simulink model "initial_setup"  (R2012b)
settings: Solver=FixedStepDiscrete  StartTime=0.0  StopTime=inf  FixedStep=sample_time  RelTol=1e-3
InitFcn:
  | init_initial_setup;
values from neighbouring files (symbols this model uses):
  fcut_unwrap = 50    [init_initial_setup.m]
  fcut_velocity = 100    [init_initial_setup.m]
  sample_time = 1/update_freq    (= 0.001)    [init_initial_setup.m]
undefined symbols (not defined in the file or in its folder): A_angle_h, A_angle_k, A_angle_lat, angle_midpoint_h, angle_midpoint_k, angle_midpoint_lat, BOOM_MAX_ENCODER_TICKS, BOOM_PITCH_CAL_VALUE_RAD, BOOM_PITCH_CAL_VALUE_TICKS, BOOM_PITCH_ENCODER_RAD_PER_TICK, BOOM_ROLL_CAL_VALUE_RAD, BOOM_ROLL_CAL_VALUE_TICKS, BOOM_ROLL_ENCODER_RAD_PER_TICK, BOOM_YAW_ENCODER_RAD_PER_TICK, control_start_time, HIP_ABS_ENCODER_RAD_PER_TICK, HIP_INC_ENCODER_RAD_PER_TICK, HIP_INC_MAX_ENCODER_TICKS, k_leg_spring, kd_h_sine_walk, kd_k_sine_walk, kd_lat, kd_sea_position, kd_sea_torque, kd_velocity, kp_h_sine_walk, kp_k_sine_walk, kp_lat, kp_sea_position, kp_sea_torque, kp_velocity, LEFT_HIP_CALIB_POS, LEFT_HIP_CALIB_VAL, LEFT_MOTOR_HIP_DIRECTION, LEG1_LEG_A_CALIB_VAL, LEG1_LEG_A_RAD_PER_CNT, LEG1_LEG_B_CALIB_VAL, LEG1_LEG_B_RAD_PER_CNT, LEG1_MOTOR_A_DIRECTION, LEG1_MOTOR_B_DIRECTION, LEG1_TRAN_A_CALIB_VAL, LEG1_TRAN_A_RAD_PER_CNT, LEG1_TRAN_B_CALIB_VAL, LEG1_TRAN_B_RAD_PER_CNT, LEG2_LEG_A_CALIB_VAL, LEG2_LEG_A_RAD_PER_CNT, LEG2_LEG_B_CALIB_VAL, LEG2_LEG_B_RAD_PER_CNT, LEG2_MOTOR_A_DIRECTION, LEG2_MOTOR_B_DIRECTION, LEG2_TRAN_A_CALIB_VAL, LEG2_TRAN_A_RAD_PER_CNT, LEG2_TRAN_B_CALIB_VAL, LEG2_TRAN_B_RAD_PER_CNT, LEG_A_CALIB_LOC, LEG_B_CALIB_LOC, LEG_MTR_GEAR_RATIO, LEG_MTR_MAX_TORQUE, LEG_MTR_MAX_VELOCITY, MTR_HIP_MAX_CURRENT ... (+10)
libraries: xpcethercatlib x160, simulink x34, dspswit3 x1
(part 4 of 4)

== system initial_setup/Simple Sinusoidal Motion/SEA Controllers (Left Leg)/SEA Controller (Velocity) front/PID/filtered_derivative ==
  x : Inport
  Gain1 : Gain  Gain=1/sample_time
  difference : simulink/Discrete/Difference  ICPrevInput=0.0  InputProcessing=Inherited  OutMin=[]  OutMax=[]  OutDataType=fixdt(1, 16)  OutScaling=2^-10  DoSatur=off
  single_pole_filter : DiscreteTransferFcn  Numerator=[(1-exp(-2*pi*fcut_velocity*sample_time)) 0]  Denominator=[1 -exp(-2*pi*fcut_velocity*sample_time)]  SampleTime=sample_time
  dx/dt : Outport
  wires:
  Gain1/1 -> single_pole_filter/1
  difference/1 -> Gain1/1
  single_pole_filter/1 -> dx/dt/1
  x/1 -> difference/1

== system initial_setup/Simple Sinusoidal Motion/SEA Controllers (Right Leg)/SEA Controller (Position) back/Position PD/filtered_derivative ==
  x : Inport
  Gain1 : Gain  Gain=1/sample_time
  difference : simulink/Discrete/Difference  ICPrevInput=0.0  InputProcessing=Inherited  OutMin=[]  OutMax=[]  OutDataType=fixdt(1, 16)  OutScaling=2^-10  DoSatur=off
  single_pole_filter : DiscreteTransferFcn  Numerator=[(1-exp(-2*pi*fcut_velocity*sample_time)) 0]  Denominator=[1 -exp(-2*pi*fcut_velocity*sample_time)]  SampleTime=sample_time
  dx/dt : Outport
  wires:
  Gain1/1 -> single_pole_filter/1
  difference/1 -> Gain1/1
  single_pole_filter/1 -> dx/dt/1
  x/1 -> difference/1

== system initial_setup/Simple Sinusoidal Motion/SEA Controllers (Right Leg)/SEA Controller (Position) front/Position PD/filtered_derivative ==
  x : Inport
  Gain1 : Gain  Gain=1/sample_time
  difference : simulink/Discrete/Difference  ICPrevInput=0.0  InputProcessing=Inherited  OutMin=[]  OutMax=[]  OutDataType=fixdt(1, 16)  OutScaling=2^-10  DoSatur=off
  single_pole_filter : DiscreteTransferFcn  Numerator=[(1-exp(-2*pi*fcut_velocity*sample_time)) 0]  Denominator=[1 -exp(-2*pi*fcut_velocity*sample_time)]  SampleTime=sample_time
  dx/dt : Outport
  wires:
  Gain1/1 -> single_pole_filter/1
  difference/1 -> Gain1/1
  single_pole_filter/1 -> dx/dt/1
  x/1 -> difference/1

== system initial_setup/Simple Sinusoidal Motion/SEA Controllers (Right Leg)/SEA Controller (Velocity) back/PD/filtered_derivative ==
  x : Inport
  Gain1 : Gain  Gain=1/sample_time
  difference : simulink/Discrete/Difference  ICPrevInput=0.0  InputProcessing=Inherited  OutMin=[]  OutMax=[]  OutDataType=fixdt(1, 16)  OutScaling=2^-10  DoSatur=off
  single_pole_filter : DiscreteTransferFcn  Numerator=[(1-exp(-2*pi*fcut_velocity*sample_time)) 0]  Denominator=[1 -exp(-2*pi*fcut_velocity*sample_time)]  SampleTime=sample_time
  dx/dt : Outport
  wires:
  Gain1/1 -> single_pole_filter/1
  difference/1 -> Gain1/1
  single_pole_filter/1 -> dx/dt/1
  x/1 -> difference/1

== system initial_setup/Simple Sinusoidal Motion/SEA Controllers (Right Leg)/SEA Controller (Velocity) back/PID/filtered_derivative ==
  x : Inport
  Gain1 : Gain  Gain=1/sample_time
  difference : simulink/Discrete/Difference  ICPrevInput=0.0  InputProcessing=Inherited  OutMin=[]  OutMax=[]  OutDataType=fixdt(1, 16)  OutScaling=2^-10  DoSatur=off
  single_pole_filter : DiscreteTransferFcn  Numerator=[(1-exp(-2*pi*fcut_velocity*sample_time)) 0]  Denominator=[1 -exp(-2*pi*fcut_velocity*sample_time)]  SampleTime=sample_time
  dx/dt : Outport
  wires:
  Gain1/1 -> single_pole_filter/1
  difference/1 -> Gain1/1
  single_pole_filter/1 -> dx/dt/1
  x/1 -> difference/1

== system initial_setup/Simple Sinusoidal Motion/SEA Controllers (Right Leg)/SEA Controller (Velocity) front/PD/filtered_derivative ==
  x : Inport
  Gain1 : Gain  Gain=1/sample_time
  difference : simulink/Discrete/Difference  ICPrevInput=0.0  InputProcessing=Inherited  OutMin=[]  OutMax=[]  OutDataType=fixdt(1, 16)  OutScaling=2^-10  DoSatur=off
  single_pole_filter : DiscreteTransferFcn  Numerator=[(1-exp(-2*pi*fcut_velocity*sample_time)) 0]  Denominator=[1 -exp(-2*pi*fcut_velocity*sample_time)]  SampleTime=sample_time
  dx/dt : Outport
  wires:
  x/1 -> difference/1
  single_pole_filter/1 -> dx/dt/1
  difference/1 -> Gain1/1
  Gain1/1 -> single_pole_filter/1

== system initial_setup/Simple Sinusoidal Motion/SEA Controllers (Right Leg)/SEA Controller (Velocity) front/PID/filtered_derivative ==
  x : Inport
  Gain1 : Gain  Gain=1/sample_time
  difference : simulink/Discrete/Difference  ICPrevInput=0.0  InputProcessing=Inherited  OutMin=[]  OutMax=[]  OutDataType=fixdt(1, 16)  OutScaling=2^-10  DoSatur=off
  single_pole_filter : DiscreteTransferFcn  Numerator=[(1-exp(-2*pi*fcut_velocity*sample_time)) 0]  Denominator=[1 -exp(-2*pi*fcut_velocity*sample_time)]  SampleTime=sample_time
  dx/dt : Outport
  wires:
  x/1 -> difference/1
  single_pole_filter/1 -> dx/dt/1
  difference/1 -> Gain1/1
  Gain1/1 -> single_pole_filter/1

== matlab function initial_setup/DAQ/Supervisory ==
  data: u input; backLAmp1 output; backLAmp2 output; frontLAmp1 output; frontLAmp2 output; backRAmp1 output; backRAmp2 output; frontRAmp1 output; frontRAmp2 output; backLError output; frontLError output; backRError output; frontRError output; backLMotorV output; backLLogicV output; frontLMotorV output; frontLLogicV output; backRMotorV output; backRLogicV output; frontRMotorV output; frontRLogicV output; frontLTemp0 output; frontLTemp1 output; frontLTemp2 output; frontLTemp3 output; frontLTemp4 output; frontLTemp5 output; backLTemp0 output; backLTemp1 output; backLTemp2 output; backLTemp3 output; backLTemp4 output; backLTemp5 output
function [backLAmp1, backLAmp2, frontLAmp1, frontLAmp2, backRAmp1, ....
    backRAmp2, frontRAmp1, frontRAmp2, backLError, frontLError, ...
    backRError, frontRError, backLMotorV, backLLogicV, frontLMotorV, ...
    frontLLogicV, backRMotorV, backRLogicV, frontRMotorV, frontRLogicV,...
    frontLTemp0, frontLTemp1, frontLTemp2, frontLTemp3, frontLTemp4,...
    frontLTemp5, backLTemp0, backLTemp1, backLTemp2, backLTemp3, ...
    backLTemp4, backLTemp5]    = fcn(u)

 % amplifiers
 backRAmp1 = u(17);
 backRAmp2 = u(18);
 frontRAmp1 = u(37);
 frontRAmp2 = u(38);
 backLAmp1 = u(57);
 backLAmp2 = u(58);
 frontLAmp1 = u(77);
 frontLAmp2 = u(78);
 
 % error flags
 backRError = u(4);
 frontRError = u(24);
 backLError = u(44);
 frontLError = u(64);
 
 % voltages
  backRMotorV = u(9);
  backRLogicV = u(10);
  frontRMotorV = u(29);
  frontRLogicV = u(30);
  backLMotorV = u(49);
  backLLogicV = u(50);
  frontLMotorV = u(69);
  frontLLogicV = u(70);
  
  % temperature
  frontLTemp0 = u(71);
  frontLTemp1 = u(72);
  frontLTemp2 = u(73);
  frontLTemp3 = u(74);
  frontLTemp4 = u(75);
  frontLTemp5 = u(76);
  backLTemp0 = u(51);
  backLTemp1 = u(52);
  backLTemp2 = u(53);
  backLTemp3 = u(54);
  backLTemp4 = u(55);
  backLTemp5 = u(56);
end
